simulink model "PID"  (R2020b)
settings: Solver=VariableStepAuto  StartTime=0.0  StopTime=10.0  RelTol=1e-3
undefined symbols (not defined in the file): Ki, Kp, Ts
settings Model: Creator=admin  LastModifiedBy=admin

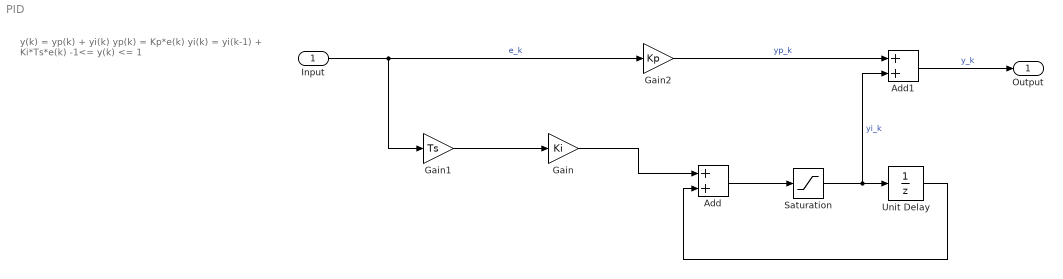
== system PID ==
  note: y(k) = yp(k) + yi(k)
      |
      | yp(k) = Kp*e(k)
      |
      | yi(k) = yi(k-1) + Ki*Ts*e(k)
      |
      | -1<= y(k) <= 1
  Input : Inport
  Add : Sum
  Add1 : Sum
  Gain : Gain  Gain=Ki
  Gain1 : Gain  Gain=Ts
  Gain2 : Gain  Gain=Kp
  Saturation : Saturate  UpperLimit=1  LowerLimit=-1
  Unit Delay : UnitDelay  SampleTime=-1  HasFrameUpgradeWarning=on
  Output : Outport
  wires:
  Gain1/1 -> Gain/1
  Gain/1 -> Add/1
  Unit Delay/1 -> Add/2
  Gain2/1 -> Add1/1  "yp_k"
  Input/1 -> Gain1/1, Gain2/1  "e_k"
  Add/1 -> Saturation/1
  Saturation/1 -> Add1/2, Unit Delay/1  "yi_k"
  Add1/1 -> Output/1  "y_k"
